simulink model "SatDinModel_3_CEK"  (Simulink 7.7)
settings: Solver=ode45  StartTime=0.0  StopTime=7200  FixedStep=1  RelTol=1e-3
undefined symbols (not defined in the file or in its folder): coe2rv, rv2OrbFrame
libraries: aerolibconvert2 x4, aerolibanimutils x1, aerolibanim x1, vrlib x1
settings Model: Creator=Ridanto  LastModifiedBy=Ridanto  BufferReuse=off
settings OptimizationCC: BufferReuse=off  InitFltsAndDblsToZero=on
settings DebuggingCC: SaveWithParameterizedLinksMsg=none  SignalResolutionControl=TryResolveAllWithWarning  MultiTaskDSMMsg=warning  MultiTaskCondExecSysMsg=none  StrictBusMsg=Warning
settings SFSimCC: SimParseCustomCode=off
settings RTWCC: IncludeERTFirstTime=on
settings GRTTargetCC: TargetFcnLib=ansi_tfl_tmw.mat

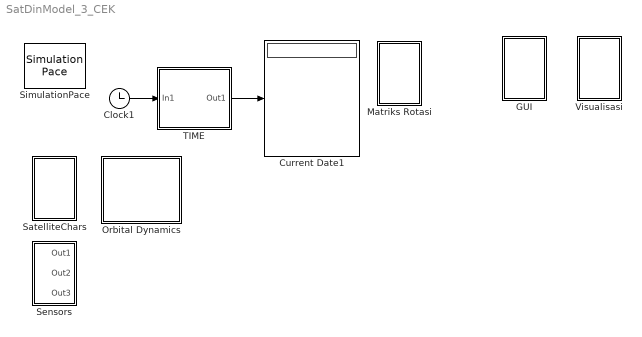
== system SatDinModel_3_CEK ==
  Clock1 : Clock
      settings: Decimation=10
  Current Date1 : Display
  GUI : Subsystem
  Matriks Rotasi : Subsystem
  Orbital Dynamics : Subsystem
  SatelliteChars : Subsystem
  Sensors : Subsystem
  SimulationPace : aerolibanimutils/Simulation Pace  SimulationPace=60  SleepMode=MATLAB Thread  OutputPaceError=off  SampleTime=1/30
      settings: AttributesFormatString=%<SimulationPace> sec/sec
  TIME : Subsystem
  Visualisasi : Subsystem
  wires:
  Clock1/1 -> TIME/1(In1)
  TIME/1(Out1) -> Current Date1/1

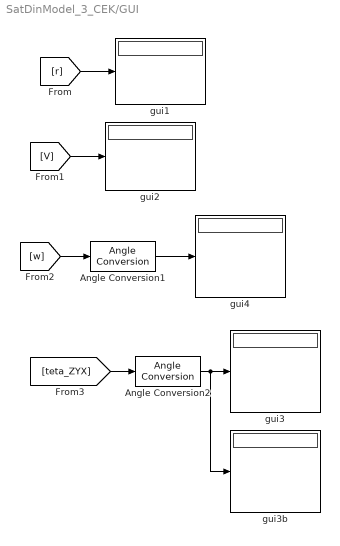
== system SatDinModel_3_CEK/GUI ==
  Angle Conversion1 : aerolibconvert2/Angle Conversion  SystemSampleTime=-1  IU=rad  OU=deg
  Angle Conversion2 : aerolibconvert2/Angle Conversion  SystemSampleTime=-1  IU=rad  OU=deg
  gui{1..4} (4 alike) : Display
  gui3b : Display
  wires:
  [r] -> gui1/1
  [V] -> gui2/1
  Angle Conversion1/1 -> gui4/1
  [w] -> Angle Conversion1/1
  [teta_ZYX] -> Angle Conversion2/1
  Angle Conversion2/1 -> gui3/1, gui3b/1

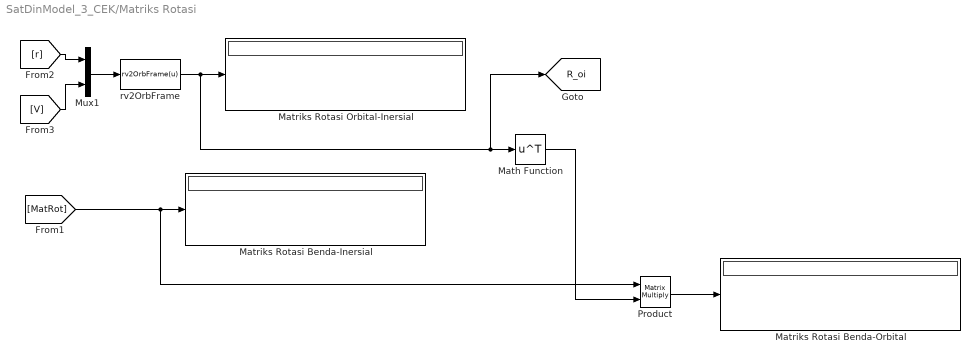
== system SatDinModel_3_CEK/Matriks Rotasi ==
  Math Function : Math  Operator=transpose  SaturateOnIntegerOverflow=on
  Matriks Rotasi Benda-Inersial : Display
  Matriks Rotasi Benda-Orbital : Display
  Matriks Rotasi Orbital-Inersial : Display
  Mux1 : Mux  Inputs=2
  Product : Product  Multiplication=Matrix(*)  RndMeth=Zero
  rv2OrbFrame : MATLABFcn  MATLABFcn=rv2OrbFrame(u)  Output1D=off
  tag scope: R_oi=global
  wires:
  [r] -> Mux1/1
  [V] -> Mux1/2
  Mux1/1 -> rv2OrbFrame/1
  rv2OrbFrame/1 -> Matriks Rotasi Orbital-Inersial/1, Math Function/1, [R_oi]
  [MatRot] -> Matriks Rotasi Benda-Inersial/1, Product/1
  Math Function/1 -> Product/2
  Product/1 -> Matriks Rotasi Benda-Orbital/1

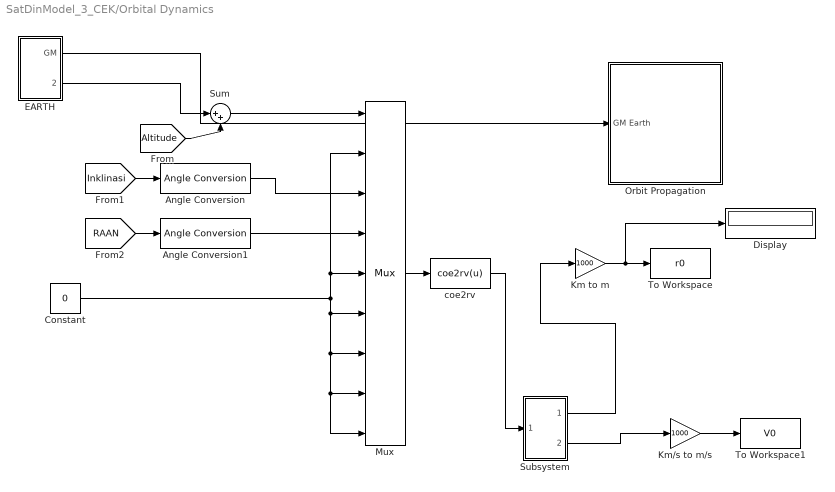
== system SatDinModel_3_CEK/Orbital Dynamics ==
  Angle Conversion : aerolibconvert2/Angle Conversion  SystemSampleTime=-1  IU=deg  OU=rad
  Angle Conversion1 : aerolibconvert2/Angle Conversion  SystemSampleTime=-1  IU=deg  OU=rad
  Constant : Constant  Value=0
  Display : Display
  EARTH : Subsystem
  Km to m : Gain  Gain=1000
  Km/s to m/s : Gain  Gain=1000
  Mux : Mux  Inputs=9
  Orbit Propagation : Subsystem
  Subsystem : Subsystem
  Sum : Sum  Inputs=|++
  To Workspace : ToWorkspace  VariableName=r0  SampleTime=-1  SaveFormat=Structure
  To Workspace1 : ToWorkspace  VariableName=V0  SampleTime=-1  SaveFormat=Structure
  coe2rv : MATLABFcn  MATLABFcn=coe2rv(u)
  wires:
  EARTH/1(GM) -> Orbit Propagation/1(GM Earth)
  EARTH/2(Radius) -> Sum/1
  Angle Conversion/1 -> Mux/3
  Sum/1 -> Mux/1
  Angle Conversion1/1 -> Mux/4
  Mux/1 -> coe2rv/1
  Constant/1 -> Mux/2, Mux/5, Mux/6, Mux/7, Mux/8, Mux/9
  [Altitude] -> Sum/2
  [Inklinasi] -> Angle Conversion/1
  [RAAN] -> Angle Conversion1/1
  Km to m/1 -> To Workspace/1, Display/1
  Km/s to m/s/1 -> To Workspace1/1
  coe2rv/1 -> Subsystem/1(In1)
  Subsystem/2(Out2) -> Km/s to m/s/1
  Subsystem/1(Out1) -> Km to m/1

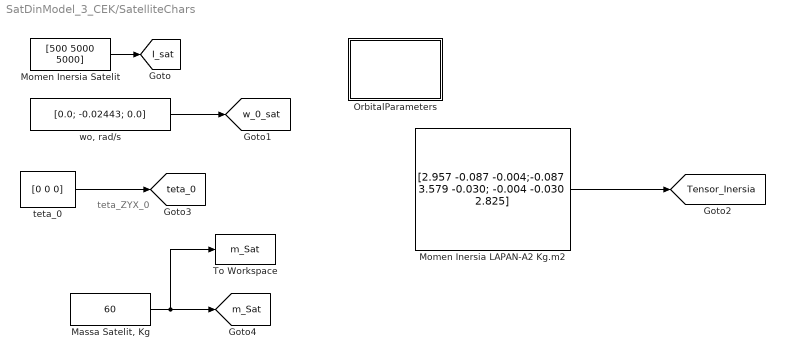
== system SatDinModel_3_CEK/SatelliteChars ==
  note: teta_ZYX_0
  "Massa Satelit, Kg" : Constant  Value=60
  Momen Inersia LAPAN-A2 Kg.m2 : Constant  Value=[2.957 -0.087 -0.004;-0.087 3.579 -0.030; -0.004 -0.030 2.825]
  Momen Inersia Satelit : Constant  Value=[500 5000 5000]
  OrbitalParameters : Subsystem
  To Workspace : ToWorkspace  VariableName=m_Sat  SampleTime=-1  SaveFormat=Structure
  teta_0 : Constant  Value=[0 0 0]
  "wo, rad/s" : Constant  Value=[0.0; -0.02443; 0.0]
  tag scope: I_sat=global, Tensor_Inersia=global, m_Sat=global, teta_0=global, w_0_sat=global
  wires:
  Momen Inersia Satelit/1 -> [I_sat]
  "wo, rad/s"/1 -> [w_0_sat]
  teta_0/1 -> [teta_0]
  Momen Inersia LAPAN-A2 Kg.m2/1 -> [Tensor_Inersia]
  "Massa Satelit, Kg"/1 -> [m_Sat], To Workspace/1

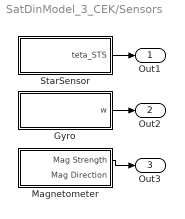
== system SatDinModel_3_CEK/Sensors ==
  Gyro : Subsystem
  Magnetometer : Subsystem
  StarSensor : Subsystem
  Out1 : Outport
  Out2 : Outport  Port=2
  Out3 : Outport  Port=3
  wires:
  StarSensor/1(teta_STS) -> Out1/1
  Gyro/1(w) -> Out2/1
  Magnetometer/1(Mag Strength) -> Out3/1

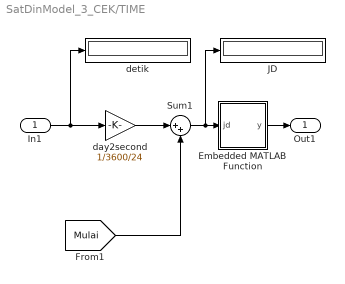
== system SatDinModel_3_CEK/TIME ==
  In1 : Inport
  Embedded MATLAB Function : Stateflow chart  TreatAsAtomicUnit=on
  JD : Display
  Sum1 : Sum  Inputs=|++
  day2second : Gain  Gain=1/3600/24
  detik : Display
  Out1 : Outport
  wires:
  In1/1 -> detik/1, day2second/1
  day2second/1 -> Sum1/1
  Sum1/1 -> Embedded MATLAB Function/1(jd), JD/1
  Embedded MATLAB Function/1(y) -> Out1/1
  [Mulai] -> Sum1/2

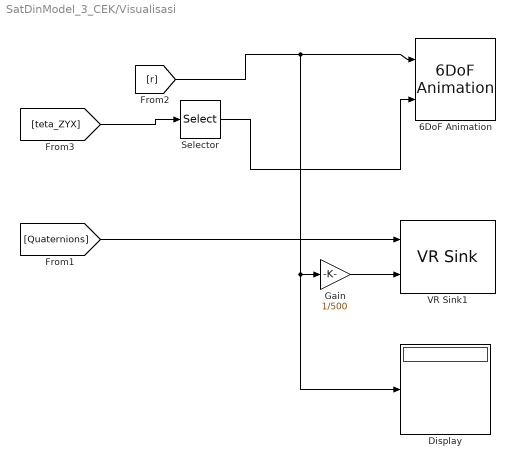
== system SatDinModel_3_CEK/Visualisasi ==
  6DoF Animation : aerolibanim/6DoF Animation  SystemSampleTime=-1  u1=[-10000 10000 -10000 10000 -10000 10000]  u2=2  u3=2000  u4=[0 0 0]  u5=Fixed position  u6=[60000 120000 60000]  u7=10  u8=on
      link override Animation S-Function: FunctionName=sSATanim3
  Display : Display
  Gain : Gain  Gain=1/500
  Selector : Selector  InputPortWidth=3  IndexOptions=Index vector (dialog)  Indices=[3 2 1]  OutputSizes=1
  VR Sink1 : vrlib/VR Sink  SampleTime=20  ViewEnable=on  RemoteChange=off  RemoteView=on  FieldsWritten=satelit.rotation.4.1.1.double#satelit.translation.3.1.1.double  WorldFileName=vrattsat.WRL  AutoView=off  VideoDimensions=[]
  wires:
  [teta_ZYX] -> Selector/1
  [r] -> 6DoF Animation/1, Display/1, Gain/1
  Selector/1 -> 6DoF Animation/2
  [Quaternions] -> VR Sink1/1
  Gain/1 -> VR Sink1/2

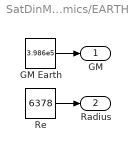
== system SatDinModel_3_CEK/Orbital Dynamics/EARTH ==
  GM Earth : Constant  Value=3.986e5
  Re : Constant  Value=6378
  GM : Outport
  Radius : Outport  Port=2
  wires:
  GM Earth/1 -> GM/1
  Re/1 -> Radius/1

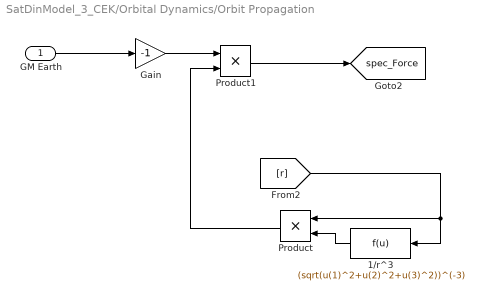
== system SatDinModel_3_CEK/Orbital Dynamics/Orbit Propagation ==
  GM Earth : Inport
  1/r^3 : Fcn  Expr=(sqrt(u(1)^2+u(2)^2+u(3)^2))^(-3)
  Gain : Gain  Gain=-1
  Product : Product  RndMeth=Zero
  Product1 : Product  RndMeth=Zero
  tag scope: spec_Force=global
  wires:
  GM Earth/1 -> Gain/1
  1/r^3/1 -> Product/2
  Product/1 -> Product1/2
  Gain/1 -> Product1/1
  Product1/1 -> [spec_Force]
  [r] -> 1/r^3/1, Product/1

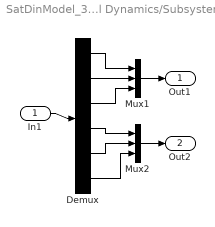
== system SatDinModel_3_CEK/Orbital Dynamics/Subsystem ==
  In1 : Inport
  Demux : Demux  Outputs=6
  Mux1 : Mux  Inputs=3
  Mux2 : Mux  Inputs=3
  Out1 : Outport
  Out2 : Outport  Port=2
  wires:
  Demux/1 -> Mux1/1
  Demux/2 -> Mux1/2
  Demux/3 -> Mux1/3
  Demux/4 -> Mux2/1
  Demux/5 -> Mux2/2
  Demux/6 -> Mux2/3
  Mux1/1 -> Out1/1
  In1/1 -> Demux/1
  Mux2/1 -> Out2/1

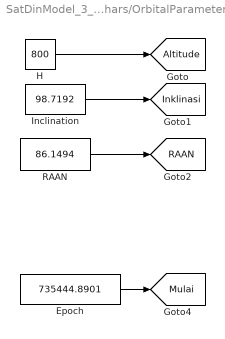
== system SatDinModel_3_CEK/SatelliteChars/OrbitalParameters ==
  Epoch : Constant  Value=735444.8901
  H : Constant  Value=800
  Inclination : Constant  Value=98.7192
  RAAN : Constant  Value=86.1494
  tag scope: Altitude=global, Inklinasi=global, Mulai=global, RAAN=global
  wires:
  H/1 -> [Altitude]
  Inclination/1 -> [Inklinasi]
  RAAN/1 -> [RAAN]
  Epoch/1 -> [Mulai]

== system SatDinModel_3_CEK/Sensors/Gyro ==
  w : Outport

== system SatDinModel_3_CEK/Sensors/Magnetometer ==
  Mag Strength : Outport
  Mag Direction : Outport  Port=2

== system SatDinModel_3_CEK/Sensors/StarSensor ==
  teta_STS : Outport

== matlab function TIME/Embedded MATLAB Function ==
  data: jd input double; y output double
function y = fcn(jd)
%#eml

 % ----------------- find year and days of the year ---------------
     temp   = jd-2415019.5+1721044.5+14;
     tu     = temp / 365.25;
     year   = 1900 + floor( tu );
     leapyrs= floor( ( year-1901 )*0.25 );
%     days   = temp - ((year-1900)*365.0 + leapyrs ) + 0.00000000001; % nudge by 8.64x10-7 sec to get even outputs
     days   = temp - ((year-1900)*365.0 + leapyrs );

     % ------------ check for case of beginning of a year -------------
     if days < 1.0
         year   = year - 1;
         leapyrs= floor( ( year-1901 )*0.25 );
         days   = temp - ((year-1900)*365.0 + leapyrs );
       end

     % ------------------- find remaining data  -----------------------
     
     % --------------- set up array of days in month  --------------
     lmonth=[31;28;31;30;31;30;31;31;30;31;30;31];
          
     dayofyr= floor(days );

        % ----------------- find month and day of month ---------------
        if modulo(year-1900,4) == 0
            lmonth(2)= 29;
          end

        i= 1;
        inttemp= 0;
        while ( dayofyr > inttemp + lmonth(i) ) & ( i < 12 )
            inttemp= inttemp + lmonth(i);
            i= i+1;
          end

        mon= i;
        day= dayofyr - inttemp;

        % ----------------- find hours minutes and seconds ------------
        temp= (days - dayofyr )*24.0;
        hr  = fix( temp );
        temp= (temp-hr) * 60.0;
        min = fix( temp );
        sec = (temp-min) * 60.0;
%     sec= sec - 0.00000086400;


y = [year;mon;day;hr;min;sec];
